simulink library "scc"  (Simulink 8.1)
settings: Solver=ode1  StartTime=0.0  StopTime=Inf  FixedStep=0.001  RelTol=1e-3
PostLoadFcn:
  | , if any(exist('dsrtsu_mdlpostloadfcn', 'file') == [2, 3, 6]), try dsrtsu_mdlpostloadfcn('Execute', bdroot); catch fprintf('Error in PostLoadFcn (dsrtsu_mdlpostloadfcn) for model "%s":\n %s\n', bdroot, lasterr); end, end,
undefined symbols (not defined in the file or in its folder): ENUM_ACCHMISTATE_ACTIVE, ENUM_ACCHMISTATE_ERROR, ENUM_ACCHMISTATE_OFF, ENUM_ACCHMISTATE_STANDBY, ENUM_ACCSTATE_DISABLED, ENUM_ACCSTATE_HOLD, ENUM_ACCSTATE_OFF, ENUM_ACCSTATE_OVERRIDE, ENUM_ACCSTATE_SPEED, ENUM_ACCSTATE_STANDBY, ENUM_ACCSTATE_STANDSTILL, FALSE, TRUE
settings Model: DSRTSU_INTERNAL_RTI_VER=450  DSRTSU_INTERNAL_RTI_TYPE=rti1401  RTICANMMDATA=struct('GeneralSetupData',struct('modelroot','D:\ELN150201_TAIWAN\trunk\AdasDragon\software\sw_development\arch\app\acc','generalsettings',struct('filesettings',struct('destfolder',struct('Name','RTICANMM_FILES','Check',1),'buildfolder',struct('Name','.','Check',1),'AbsDestfolder',struct('Name','D:\ELN150201_TAIWAN\trunk\AdasDragon\software\sw_development\arch\app\acc\RTICANMM_FILES'),'AbsBuildfolder',struct('Name','D:\ELN150201_TAIWAN\trunk\AdasDragon\software\sw_development\arch\app\acc'))),'options',struct('addpaths',1,'rmpaths',1,'addtrcexclusion',logical(1),'cannavigator',struct('checkmonitoring',0),'show_usrtrc',0,'use_usrtrc',0),'advanced',struct('options',[1 1 1 1 1 1 1 1 1 1 1 1 1 1 1 1 1 1 1 1 1 1 1 1 1 1 1 1 1 1 1 1 1 1 1 1 1 1 1 1 1 1 1 1 1 1 1 1 1 1 1 1 1 1 1 1 1 1 1 1 1 1 1 1 1 1 1 1 1 1 1 1 1 1 1 1 1 1 1 1 1 1 1 1 1 1 1 1 1 1 1 1 1 1 1 1 1 1 1 1]),'MPSetup',{{}},'modelname','scc','block','scc'))  DSRTSU_INTERNAL_RTIFPGA=40  Creator=AT015411  LastModifiedBy=AT015555

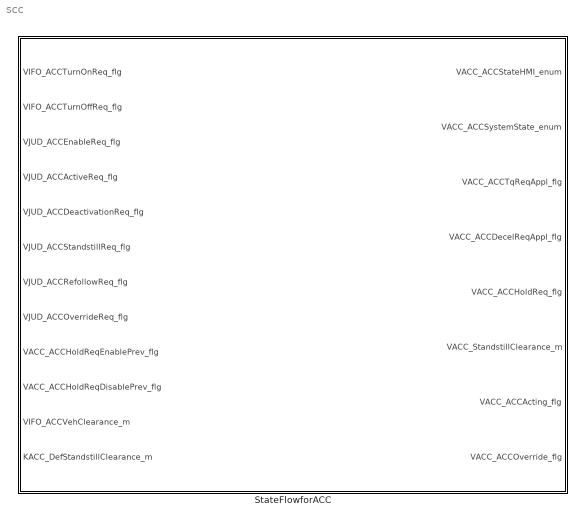
== system scc ==
  StateFlowforACC : Stateflow chart  TreatAsAtomicUnit=on

== stateflow chart StateFlowforACC ==
  state DISABLED
    en:
    VACC_ACCSystemState_enum = ENUM_ACCSTATE_DISABLED;
    VACC_ACCStateHMI_enum = ENUM_ACCHMISTATE_ERROR;
    VACC_ACCTqReqAppl_flg=FALSE;
    VACC_ACCDecelReqAppl_flg=FALSE;
    VACC_ACCActing_flg=FALSE;
    VACC_ACCHoldReq_flg = FALSE;
    VACC_ACCOverride_flg=FALSE;
    VACC_StandstillClearance_m=KACC_DefStandstillClearance_m;
  state ENABLED
    state OFF
      en:
      VACC_ACCSystemState_enum = ENUM_ACCSTATE_OFF;
      VACC_ACCStateHMI_enum = ENUM_ACCHMISTATE_OFF;
    state STANDBY
      en:
      VACC_ACCSystemState_enum = ENUM_ACCSTATE_STANDBY;
      VACC_ACCStateHMI_enum = ENUM_ACCHMISTATE_STANDBY;
    state ACTIVE
      en:
      VACC_ACCStateHMI_enum = ENUM_ACCHMISTATE_ACTIVE;
      VACC_ACCActing_flg = TRUE;
      VACC_ACCTqReqAppl_flg=TRUE;
      VACC_ACCDecelReqAppl_flg=TRUE;
      ex:
      VACC_ACCActing_flg = FALSE;
      VACC_ACCTqReqAppl_flg=FALSE;
      VACC_ACCDecelReqAppl_flg=FALSE;
      VACC_ACCHoldReq_flg = FALSE;
      state SPEED_MODE
        en:
        VACC_ACCSystemState_enum = ENUM_ACCSTATE_SPEED;
        VACC_ACCHoldReq_flg = FALSE;
      state STANDSTILL
        en:
        VACC_ACCSystemState_enum = ENUM_ACCSTATE_STANDSTILL;
        VACC_ACCTqReqAppl_flg=FALSE;
        VACC_StandstillClearance_m=VIFO_ACCVehClearance_m;
        ex:
        VACC_ACCTqReqAppl_flg=TRUE;
        VACC_StandstillClearance_m=KACC_DefStandstillClearance_m;
      state DRIVER_OVERRIDE
        en:
        VACC_ACCSystemState_enum = ENUM_ACCSTATE_OVERRIDE;
        VACC_ACCOverride_flg=TRUE;
        VACC_ACCTqReqAppl_flg=FALSE;
        VACC_ACCDecelReqAppl_flg=FALSE;
        ex:
        VACC_ACCOverride_flg=FALSE;
        VACC_ACCTqReqAppl_flg=TRUE;
        VACC_ACCDecelReqAppl_flg=TRUE;
      state HOLD
        en:
        VACC_ACCSystemState_enum = ENUM_ACCSTATE_HOLD;
        VACC_ACCHoldReq_flg= TRUE;
      (default) -> SPEED_MODE
      SPEED_MODE -> HOLD [order 2] : [VACC_ACCHoldReqEnablePrev_flg == TRUE]
      HOLD -> STANDSTILL [order 1] : [VJUD_ACCStandstillReq_flg == TRUE]
      HOLD -> SPEED_MODE [order 2] : [VACC_ACCHoldReqDisablePrev_flg == TRUE]
      STANDSTILL -> SPEED_MODE : [VJUD_ACCRefollowReq_flg == TRUE]
      SPEED_MODE -> (junction 18) [order 1]
      (junction 17) -> SPEED_MODE
      DRIVER_OVERRIDE -> (junction 17) : [VJUD_ACCOverrideReq_flg == FALSE]
      (junction 18) -> DRIVER_OVERRIDE : [VJUD_ACCOverrideReq_flg == TRUE]
    (default) -> OFF
    OFF -> STANDBY : [VIFO_ACCTurnOnReq_flg == TRUE]
    STANDBY -> ACTIVE [order 2] : [VJUD_ACCActiveReq_flg == TRUE]
    STANDBY -> OFF [order 1] : [VIFO_ACCTurnOffReq_flg == TRUE]
    ACTIVE -> STANDBY : [VJUD_ACCDeactivationReq_flg == TRUE]
  (default) -> DISABLED
  DISABLED -> ENABLED : [VJUD_ACCEnableReq_flg == TRUE]
  ENABLED -> DISABLED : [VJUD_ACCEnableReq_flg == FALSE]
  data: VACC_ACCStateHMI_enum output uint8; VACC_ACCSystemState_enum output uint8; ENUM_ACCSTATE_DISABLED parameter uint8; ENUM_ACCSTATE_OFF parameter uint8; ENUM_ACCSTATE_STANDBY parameter uint8; ENUM_ACCSTATE_SPEED parameter uint8; ENUM_ACCSTATE_STANDSTILL parameter uint8; ENUM_ACCSTATE_OVERRIDE parameter uint8; ENUM_ACCHMISTATE_OFF parameter uint8; ENUM_ACCHMISTATE_STANDBY parameter uint8; ENUM_ACCHMISTATE_ACTIVE parameter uint8; VIFO_ACCTurnOnReq_flg input boolean; VIFO_ACCTurnOffReq_flg input boolean; VJUD_ACCEnableReq_flg input boolean; TRUE parameter boolean; FALSE parameter boolean; VJUD_ACCActiveReq_flg input boolean; VJUD_ACCDeactivationReq_flg input boolean; VJUD_ACCStandstillReq_flg input boolean; VJUD_ACCRefollowReq_flg input boolean; VJUD_ACCOverrideReq_flg input boolean; ENUM_ACCHMISTATE_ERROR parameter uint8; VACC_ACCTqReqAppl_flg output boolean; VACC_ACCDecelReqAppl_flg output boolean; VACC_ACCHoldReq_flg output boolean; VACC_StandstillClearance_m output single; VACC_ACCActing_flg output boolean; VACC_ACCOverride_flg output boolean; VACC_ACCHoldReqEnablePrev_flg input double; VACC_ACCHoldReqDisablePrev_flg input double; VIFO_ACCVehClearance_m input double; ENUM_ACCSTATE_HOLD parameter uint8; KACC_DefStandstillClearance_m input double
